simulink model "lab3Mod1"  (Simulink 10.2)
settings: Solver=ode45  StartTime=0.0  StopTime=20  MaxStep=.01  RelTol=1e-3  AbsTol=1e-6
libraries: simulink x1
settings Model: Creator=vise  LastModifiedBy=tuyuncheng  ExtModeTrigMode=oneshot  ExtModeArmWhenConnect=off  ExtModeAutoUpdateStatusClock=off
settings OptimizationCC: BooleanDataType=off  LifeSpan=auto
settings DebuggingCC: SaveWithParameterizedLinksMsg=none  SignalResolutionControl=TryResolveAllWithWarning  MultiTaskDSMMsg=warning  MultiTaskCondExecSysMsg=none  FcnCallInpInsideContextMsg=error  SFUnexpectedBacktrackingDiag=error  SFNoUnconditionalDefaultTransitionDiag=error  SFExecutionAtInitializationDiag=warning  ArithmeticOperatorsInVariantConditions=error
settings HardwareCC: ProdBitPerPointer=64  ProdBitPerSizeT=64  ProdBitPerPtrDiffT=64  ProdLargestAtomicFloat=Float  ProdIntDivRoundTo=Zero  ProdEndianess=LittleEndian  ProdWordSize=64  ProdHWDeviceType=Intel->x86-64 (Windows64)  TargetUnknown=on
settings SFSimCC: SimUseLocalCustomCode=on  CustomCodeUndefinedFunction=FilterOut
settings RTWCC: TemplateMakefile=grt_unix.tmf  RTWUseLocalCustomCode=on
settings CodeAppCC: StateflowObjectComments=off
settings GRTTargetCC: TargetLangStandard=C99 (ISO)
settings ConfigComp: CovSaveCumulativeToWorkspaceVar=off  CovSaveSingleToWorkspaceVar=off  CovExternalEMLEnable=on

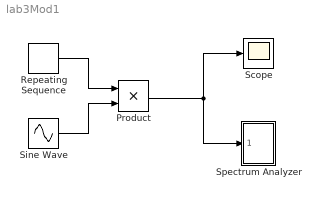
== system lab3Mod1 ==
  Product : Product  SaturateOnIntegerOverflow=on
  Repeating Sequence : simulink/Sources/Repeating Sequence  rep_seq_t=[0 1.5 3 ]  rep_seq_y=[0 1 0 ]
  Scope : Scope
  Sine Wave : Sin  Frequency=2*pi*10  SampleTime=0
  Spectrum Analyzer : Subsystem  mask(Spectrum analyzer.){N=2048, T_s=0.02, plot_period=10}
      mask prompts: N "Number of sample points:"; T_s "Sampling period (sec):"; plot_period "Plotting Period (sec):"
      mask Help: EE438 Lab utility; See Prof. Bouman.
      mask Display: plot(0,0,100,100,[14,91,91,14,14],[86,86,40,40,86],[85,82,80,79,75,67,63,60,57,53,41,36,33,27,24],[49,50,53,50,49,51,54,66,54,50,50,52,81,51,49])
  wires:
  Product/1 -> Spectrum Analyzer/1(input signal), Scope/1
  Repeating Sequence/1 -> Product/1
  Sine Wave/1 -> Product/2

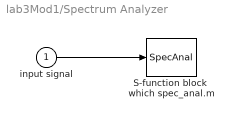
== system lab3Mod1/Spectrum Analyzer ==
  input signal : Inport
  S-function block  which spec_anal.m : S-Function  FunctionName=SpecAnal  Parameters=N,T_s,plot_period  SFunctionDeploymentMode=off  EnableBusSupport=off
  wires:
  input signal/1 -> S-function block  which spec_anal.m/1
